simulink model "State_Estimate_Tarcker"  (Simulink 8.5)
settings: Solver=ode15s  StartTime=0.0  StopTime=10.0  RelTol=1e-7
values from neighbouring files (symbols this model uses):
  A = [2.15382349002 0.214572825654 1.88950096566 -0.29867853041 0.113062196229 -1.01325242733 0.619436209547 2.86203861181 4.48591725582 -0.687413149535 3.93984391159 1.51814076611 ... (36 elements, 6x6)]    [De2.mat]    (also in main_elca.m = [   -2.1     0.3     0.5     0.9; main_elca_nonsquare.m = [-31.31 0 -2.833e4;0 -10.25 8001;1 -1 0]; main_elca_siso.m = [-31.31 0 -2.833e4;0 -10.25 8001;1 -1 0]; main_elca_siso_conference.m = [-31.31 0 -2.833e4;0 -10.25 8001;1 -1 0])
  A_aug = [    A    , zeros(n,p) ... (first row only)    [main_c.m]    (also in main_elca.m; main_elca_nonsquare.m; main_elca_siso.m; main_elca_siso_conference.m)
  Ae_aug = [ A-De*inv(eye(p)+Ked*C_tilde*De)*Ked*C_tilde*A     De*inv(eye(p)+Ked*C_tilde*De)*Kei ... (first row only)    [main_c.m]    (also in main_elca.m; main_elca_nonsquare.m; main_elca_siso.m; main_elca_siso_conference.m)
  B = [-3.59754701628 1.03900107164 -0.0588288788819 1.91030576689 -0.469593029649 2.39038747798 -2.63971513379 2.37119746965 -0.382769327239 -1.07761123079 -0.524364953631 2.34772297005 ... (18 elements, 6x3)]    [De2.mat]    (also in main_elca.m = [   1   -0.4; main_elca_nonsquare.m = [28.06 0 0]'; main_elca_siso.m = [28.06 0 0]'; main_elca_siso_conference.m = [28.06;0;0])
  B_aug = [     B ... (first row only)    [main_c.m]    (also in main_elca.m; main_elca_nonsquare.m; main_elca_siso.m; main_elca_siso_conference.m)
  Be_aug = [ De*inv(eye(p)+Ked*C_tilde*De)*Kep ... (first row only)    [main_c.m]    (also in main_elca.m; main_elca_nonsquare.m; main_elca_siso.m; main_elca_siso_conference.m)
  C_a = [De*inv(eye(p)+Ked*eta*C_tilde*De)*Ked*C_tilde*B; zeros(p,m)]    [main_c.m]
  C_aug = [ Kp*C_tilde + Kd*C_tilde*A , Ki]    [main_c.m]    (also in main_elca.m; main_elca_nonsquare.m; main_elca_siso.m; main_elca_siso_conference.m)
  C_bar = [ C_tilde  zeros(p,p)]    [main_c.m]    (also in main_elca.m; main_elca_nonsquare.m; main_elca_siso.m; main_elca_siso_conference.m)
  C_tilde = [-36.0572415255  -180.651294811  99.2348328799  38.8771414895  3.12263315375  -178.40252991; -178.74517992  -42.1890348336  178.005055961  204.417268482  61.6801181122  -104.203885973]    [De2.mat]    (also in generate_eta.m = eta*C; main_c.m = eta *C; main_elca.m = eta * C; main_elca_nonsquare.m = eta * C)
  Ce = inv(Re)*Be_aug'*inv((Ae_aug-Be_aug*Ke)')*Pe_aug    [main_c.m]
  Ce_aug = [C_tilde  zeros(p,p)]    [main_c.m]    (also in main_elca.m; main_elca_nonsquare.m; main_elca_siso.m; main_elca_siso_conference.m)
  D_aug = Kd*C_tilde*B    [main_c.m]    (also in main_elca.m; main_elca_nonsquare.m; main_elca_siso.m; main_elca_siso_conference.m)
  De = [0.318518810679  1.43017682461; 1.54076970526  2.04306947136; -0.541765795745  0.784935731305; 0.271599502383  0.685376596238; -1.34549150719  -1.13203605501; -1.47309738777  -1.64908854438]    [De2.mat]    (also in De_.mat; De_conference.mat = [-1.1479527789  -0.666890670701; 0.104874716016  0.187331024; De_term.mat; generate_De.m = randn(n,p))
  Ec = -inv(R_bar)*( ( C - D*Kc )*inv( A - B*Kc )*B - D )'*Qc    [TZOCS.m]    (also in main_c.m = -inv(R_bar)*( ( C_aug - D_aug*Kc )*inv( A_aug - B_aug*Kc )*B; main_elca.m = -inv(R_bar)*( ( C_aug - D_aug*Kc )*inv( A_aug - B_aug*Kc )*B; main_elca_nonsquare.m = -inv(R_bar)*( ( C_aug - D_aug*Kc )*inv( A_aug - B_aug*Kc )*B; main_elca_siso.m = -inv(R_bar)*( ( C_aug - D_aug*Kc )*inv( A_aug - B_aug*Kc )*B)
  Ee = -inv(Re)*( ( Ce_aug )*inv( Ae_aug - Be_aug*Ke )*Be_aug )'*Qe    [main_c.m]    (also in main_elca.m; main_elca_nonsquare.m; main_elca_siso.m; main_elca_siso_conference.m)
  Ip = [ zeros(p,n)  eye(p) ]    [main_c.m]    (also in main_elca.m; main_elca_nonsquare.m; main_elca_siso.m; main_elca_siso_conference.m)
  Ip2 = [ zeros(n,p) ; eye(p)]    [main_c.m]    (also in main_elca.m; main_elca_nonsquare.m; main_elca_siso.m; main_elca_siso_conference.m)
  Kc1 = Kc(:,1:n)    [main_c.m]    (also in main_elca.m; main_elca_nonsquare.m; main_elca_siso.m; main_elca_siso_conference.m)
  Kc2 = Kc(:,n+1:end)    [main_c.m]    (also in main_elca.m; main_elca_nonsquare.m; main_elca_siso.m; main_elca_siso_conference.m)
  Ke1 = Ke(:,1:n)    [main_c.m]    (also in main_elca.m; main_elca_nonsquare.m; main_elca_siso.m; main_elca_siso_conference.m)
  Ke2 = Ke(:,n+1:end)    [main_c.m]    (also in main_elca.m; main_elca_nonsquare.m; main_elca_siso.m; main_elca_siso_conference.m)
  n = 6    [De2.mat]    (also in disturb2.m = varargin{1}; main_c.m = size(A,1); main_elca.m = size(A,1); main_elca_nonsquare.m = size(A,1))
  p = 2    [De2.mat]    (also in TZOCS.m = size(C,1); main_c.m = size(C,1); main_elca.m = size(C,1); main_elca_nonsquare.m = size(C,1))
  xe = Xe'    [main_c.m]    (also in main_elca_siso_luenberger.m; non_main_elca_siso_luenberger.m)
  xe_aug = Xe_aug'    [main_c.m]    (also in main_elca_siso_luenberger.m; non_main_elca_siso_luenberger.m)
undefined symbols (not defined in the file or in its folder): Ke, x_aug
settings Model: Creator=koni  LastModifiedBy=Elca
settings DebuggingCC: SolverPrmCheckMsg=warning  FcnCallInpInsideContextMsg=UseLocalSettings

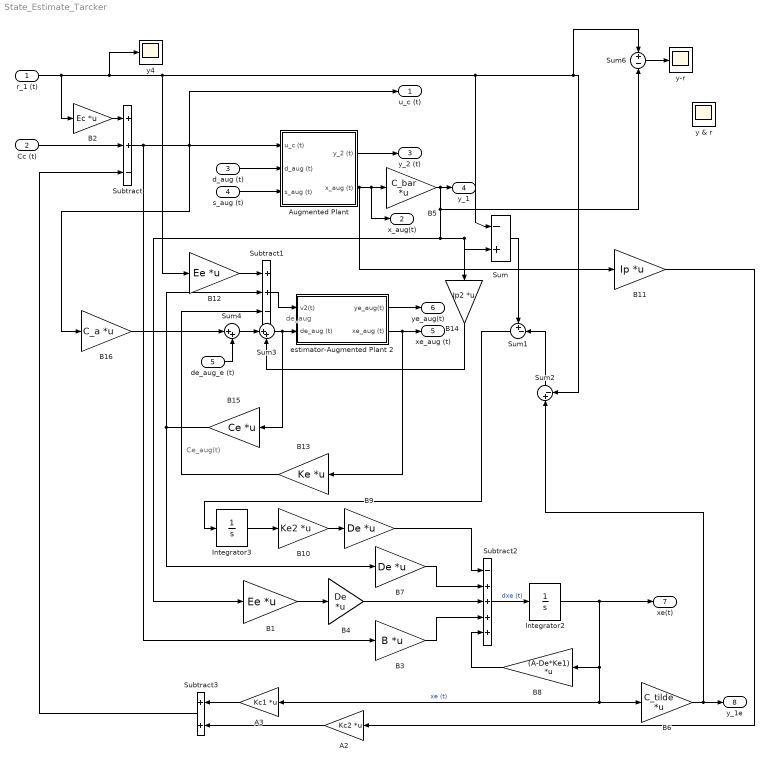
== system State_Estimate_Tarcker ==
  note: de_aug
  note: Ce_aug(t)
  r_1 (t) : Inport  PortDimensions=p
  Cc (t) : Inport  Port=2  PortDimensions=m
  d_aug (t) : Inport  Port=3  PortDimensions=n+p
  s_aug (t) : Inport  Port=4  PortDimensions=p
  de_aug_e (t) : Inport  Port=5  PortDimensions=n+p
  " Augmented Plant" : Subsystem
  A2 : Gain  Gain=Kc2  Multiplication=Matrix(K*u)
  A3 : Gain  Gain=Kc1  Multiplication=Matrix(K*u)
  B1 : Gain  Gain=Ee  Multiplication=Matrix(K*u)
  B10 : Gain  Gain=Ke2  Multiplication=Matrix(K*u)
  B11 : Gain  Gain=Ip  Multiplication=Matrix(K*u)
  B12 : Gain  Gain=Ee  Multiplication=Matrix(K*u)
  B13 : Gain  Gain=Ke  Multiplication=Matrix(K*u)
  B14 : Gain  Gain=Ip2  Multiplication=Matrix(K*u)
  B15 : Gain  Gain=Ce  Multiplication=Matrix(K*u)
  B16 : Gain  Gain=C_a  Multiplication=Matrix(K*u)
  B2 : Gain  Gain=Ec  Multiplication=Matrix(K*u)
  B3 : Gain  Gain=B  Multiplication=Matrix(K*u)
  B4 : Gain  Gain=De  Multiplication=Matrix(K*u)
  B5 : Gain  Gain=C_bar  Multiplication=Matrix(K*u)
  B6 : Gain  Gain=C_tilde  Multiplication=Matrix(K*u)
  B7 : Gain  Gain=De  Multiplication=Matrix(K*u)
  B8 : Gain  Gain=(A-De*Ke1)  Multiplication=Matrix(K*u)
  B9 : Gain  Gain=De  Multiplication=Matrix(K*u)
  Integrator2 : Integrator  InitialCondition=xe(:,1)
  Integrator3 : Integrator  InitialCondition=zeros(p,1)
  Subtract : Sum  Inputs=++-
  Subtract1 : Sum  Inputs=++-
  Subtract2 : Sum  Inputs=-++++
  Subtract3 : Sum
  Sum : Sum  Inputs=-+|
  Sum1 : Sum  Inputs=+-|
  Sum2 : Sum  Inputs=|+-
  Sum3 : Sum  Inputs=|++
  Sum4 : Sum  Inputs=|++
  Sum6 : Sum  Inputs=+-
  estimator-Augmented Plant 2 : Subsystem
  y & r : Scope
      settings: Floating=on  TickLabels=on  TimeRange=3  YMin=-2000  YMax=2000  SaveName=ScopeData5  ScrollMode=on
  y-r : Scope
      settings: TickLabels=on  TimeRange=3  YMin=-2000  YMax=750  SaveName=ScopeData6  ScrollMode=on
  y4 : Scope
      settings: TickLabels=on  ShowLegends=on  YMin=-1000  YMax=1500  SaveName=ScopeData3  ScrollMode=on
  u_c (t) : Outport  PortDimensions=m
  x_aug(t) : Outport  Port=2  PortDimensions=n+p
  y_2 (t) : Outport  Port=3  PortDimensions=p
  y_1 : Outport  Port=4  PortDimensions=p
  xe_aug (t) : Outport  Port=5  PortDimensions=n+p
  ye_aug(t) : Outport  Port=6  PortDimensions=p
  xe(t) : Outport  Port=7  PortDimensions=n
  y_1e : Outport  Port=8  PortDimensions=p
  wires:
  " Augmented Plant"/1(y_2 (t)) -> y_2 (t)/1
  Subtract/1 -> u_c (t)/1, B16/1, " Augmented Plant"/1(u_c (t)), B3/1
  B2/1 -> Subtract/1
  Cc (t)/1 -> Subtract/2
  d_aug (t)/1 -> " Augmented Plant"/2(d_aug (t))
  s_aug (t)/1 -> " Augmented Plant"/3(s_aug (t))
  B5/1 -> Sum6/2, B1/1, B14/1, Sum/2, y_1/1
  estimator-Augmented Plant 2/2(xe_aug (t)) -> xe_aug (t)/1, B13/1
  estimator-Augmented Plant 2/1(ye_aug(t)) -> ye_aug(t)/1
  Sum/1 -> Sum1/1
  Sum2/1 -> Sum1/2
  B9/1 -> Subtract2/1
  B3/1 -> Subtract2/4
  B10/1 -> B9/1
  B8/1 -> Subtract2/5
  Integrator2/1 -> B6/1, A3/1, B8/1, xe(t)/1  "xe (t)"
  Subtract2/1 -> Integrator2/1  "dxe (t)"
  B4/1 -> Subtract2/3
  B7/1 -> Subtract2/2
  Integrator3/1 -> B10/1
  B1/1 -> B4/1
  B6/1 -> Sum2/1, y_1e/1
  A2/1 -> Subtract3/2
  A3/1 -> Subtract3/1
  " Augmented Plant"/2(x_aug (t)) -> B11/1, B5/1, x_aug(t)/1
  B11/1 -> A2/1
  B13/1 -> Subtract1/3
  Subtract1/1 -> estimator-Augmented Plant 2/1(v2(t))
  B12/1 -> Subtract1/1
  Sum1/1 -> Integrator3/1
  Sum3/1 -> B15/1, estimator-Augmented Plant 2/2(de_aug (t))
  B14/1 -> Sum3/2
  B15/1 -> Subtract1/2, B7/1
  Sum4/1 -> Sum3/1
  de_aug_e (t)/1 -> Sum4/2
  B16/1 -> Sum4/1
  r_1 (t)/1 -> y4/1, Sum6/1, Sum2/2, Sum/1, B12/1, B2/1
  Subtract3/1 -> Subtract/3
  Sum6/1 -> y-r/1

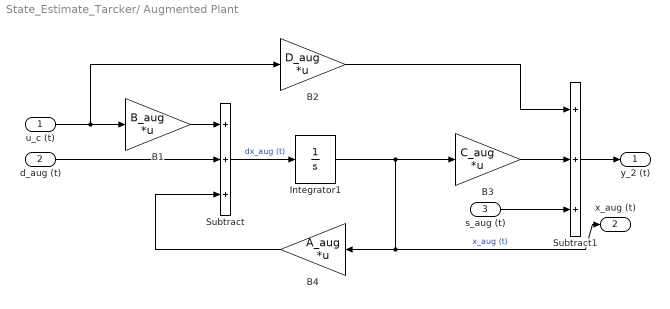
== system State_Estimate_Tarcker/ Augmented Plant ==
  u_c (t) : Inport  PortDimensions=m
  d_aug (t) : Inport  Port=2  PortDimensions=n+p
  s_aug (t) : Inport  Port=3  PortDimensions=p
  B1 : Gain  Gain=B_aug  Multiplication=Matrix(K*u)
  B2 : Gain  Gain=D_aug  Multiplication=Matrix(K*u)
  B3 : Gain  Gain=C_aug  Multiplication=Matrix(K*u)
  B4 : Gain  Gain=A_aug  Multiplication=Matrix(K*u)
  Integrator1 : Integrator  InitialCondition=x_aug(:,1)
  Subtract : Sum  Inputs=+++
  Subtract1 : Sum  Inputs=+++
  y_2 (t) : Outport  PortDimensions=p
  x_aug (t) : Outport  Port=2  PortDimensions=n+p
  wires:
  Subtract/1 -> Integrator1/1  "dx_aug (t)"
  Integrator1/1 -> x_aug (t)/1, B4/1, B3/1  "x_aug (t)"
  u_c (t)/1 -> B1/1, B2/1
  B1/1 -> Subtract/1
  Subtract1/1 -> y_2 (t)/1
  B3/1 -> Subtract1/2
  B2/1 -> Subtract1/1
  s_aug (t)/1 -> Subtract1/3
  d_aug (t)/1 -> Subtract/2
  B4/1 -> Subtract/3

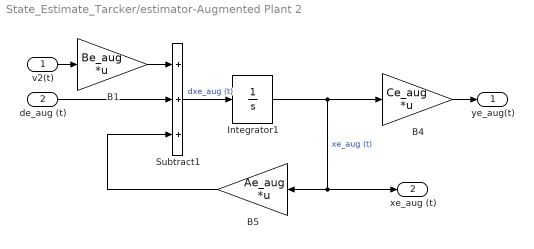
== system State_Estimate_Tarcker/estimator-Augmented Plant 2 ==
  v2(t) : Inport  PortDimensions=p
  de_aug (t) : Inport  Port=2  PortDimensions=n+p
  B1 : Gain  Gain=Be_aug  Multiplication=Matrix(K*u)
  B4 : Gain  Gain=Ce_aug  Multiplication=Matrix(K*u)
  B5 : Gain  Gain=Ae_aug  Multiplication=Matrix(K*u)
  Integrator1 : Integrator  InitialCondition=xe_aug(:,1)
  Subtract1 : Sum  Inputs=+++
  ye_aug(t) : Outport  PortDimensions=p
  xe_aug (t) : Outport  Port=2  PortDimensions=n+p
  wires:
  Subtract1/1 -> Integrator1/1  "dxe_aug (t)"
  Integrator1/1 -> xe_aug (t)/1, B5/1, B4/1  "xe_aug (t)"
  v2(t)/1 -> B1/1
  B1/1 -> Subtract1/1
  de_aug (t)/1 -> Subtract1/2
  B5/1 -> Subtract1/3
  B4/1 -> ye_aug(t)/1
